simulink model "Problem_1"  (R2020a)
settings: Solver=VariableStepAuto  StartTime=0.0  StopTime=inf  RelTol=1e-3
settings Model: Creator=Shubham Singh Rathor  LastModifiedBy=Shubham Singh Rathor
settings SolverCC: ZeroCrossAlgorithm=Adaptive
settings DebuggingCC: IgnoredZcDiagnostic=none

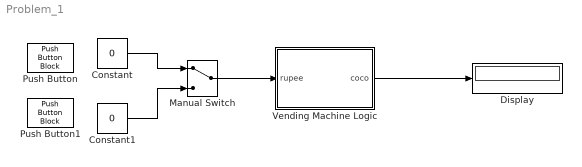
== system Problem_1 ==
  Constant : Constant  Value=0
  Constant1 : Constant  Value=0
  Display : Display
  Manual Switch : ManualSwitch
  Push Button : PushButtonBlock  ButtonText=5 rupees  OnValue=5
  Push Button1 : PushButtonBlock  ButtonText=10 rupees  OnValue=10
  Vending Machine Logic : Stateflow chart  TreatAsAtomicUnit=on
  wires:
  Vending Machine Logic/1(coco) -> Display/1
  Constant/1 -> Manual Switch/1
  Constant1/1 -> Manual Switch/2
  Manual Switch/1 -> Vending Machine Logic/1(rupee)

== stateflow chart Problem_1/Vending Machine Logic ==
  settings: stateMachineType=MEALY_MACHINE
  state Ideal_State
  state R5_State
  state R10_State
  (default) -> Ideal_State
  Ideal_State -> R5_State [order 1] : [rupee == 5]{coco = 0}
  R5_State -> Ideal_State [order 2] : [rupee == 10]{coco = 1}
  Ideal_State -> R10_State [order 2] : [rupee == 10]{coco = 0}
  R10_State -> Ideal_State [order 2] : [rupee == 5]{coco = 1}
  R5_State -> R10_State [order 1] : [rupee == 5]{coco = 0}
  R10_State -> R5_State [order 1] : [rupee == 10]{coco = 1}
  data: rupee input; coco output
